simulink model "PM"  (R2021b)
settings: Solver=VariableStepAuto  StartTime=0.0  StopTime=5  MaxStep=0.00001  RelTol=1e-3
libraries: commanapbnd3 x1
settings Model: Creator=user  LastModifiedBy=user

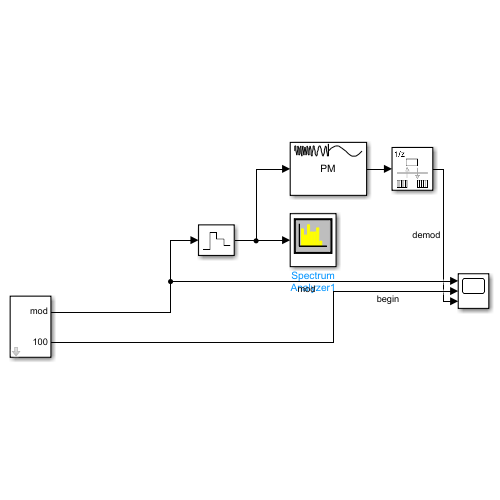
[thumbnail: Simulink's stored preview of the top-level diagram]
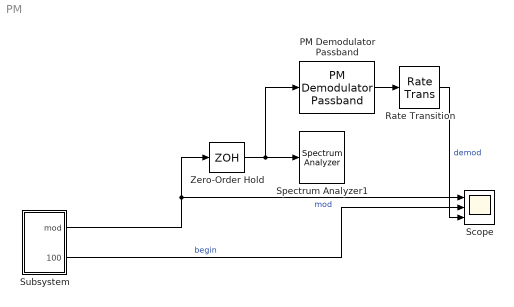
== system PM ==
  PM Demodulator Passband : commanapbnd3/PM Demodulator Passband  Fc=1000  Ph=0  Kc=pi  Ho=100
      settings: SourceProductBaseCode=CM
  Rate Transition : RateTransition
  Scope : Scope  NumInputPorts=3
  Spectrum Analyzer1 : SpectrumAnalyzer
  Subsystem : Subsystem  mask{d=2* pi}
      mask prompts: d "deviation"
  Zero-Order Hold : ZeroOrderHold  SampleTime=1e-4
  wires:
  Zero-Order Hold/1 -> PM Demodulator Passband/1, Spectrum Analyzer1/1
  PM Demodulator Passband/1 -> Rate Transition/1
  Rate Transition/1 -> Scope/3  "demod"
  Subsystem/1(mod) -> Zero-Order Hold/1, Scope/1  "mod"
  Subsystem/2(100) -> Scope/2  "begin"

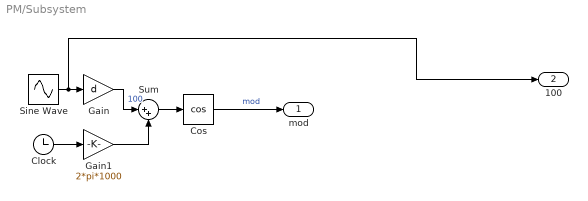
== system PM/Subsystem ==
  Clock : Clock
  Cos : Trigonometry  Operator=cos
  Gain : Gain  Gain=d
  Gain1 : Gain  Gain=2*pi*1000
  Sine Wave : Sin  Frequency=100 * 2 * pi  SampleTime=0
  Sum : Sum  Inputs=|++
  mod : Outport
  100 : Outport  Port=2
  wires:
  Cos/1 -> mod/1  "mod"
  Sum/1 -> Cos/1
  Gain1/1 -> Sum/2
  Gain/1 -> Sum/1  "100"
  Sine Wave/1 -> 100/1, Gain/1
  Clock/1 -> Gain1/1
